simulink model "EHB_MOTOR"  (R2023b)
settings: Solver=FixedStepDiscrete  StartTime=0.0  StopTime=inf  FixedStep=0.0001  RelTol=1e-3  EnableMultiTasking=on
undefined symbols (not defined in the file): CAN_EHB_VCU0x125, CAN_EHB_VCU0x126, CAN_id0x120_Data, Cos_Table, Cos_Table1, EHB_DTC_status, R, Sin_BreakPoint, Sin_BreakPoint1, Sin_Table, Sin_Table1, T
libraries: simulink x30
(part 9 of 9)

== stateflow chart EHB_MOTOR/EHB_MOTOR_PRO/INPUT/DI/Debounce7 ==
  state none
    en:cnt_0=0;
    cnt_1=0;
    none -> (junction 63)
    (junction 63) -> (junction 49) [order 1] : [input>0]
    (junction 63) -> (junction 58) [order 2]
    (junction 49) -> (junction 60)
    (junction 58) -> (junction 62) [order 1] : [cnt_0>=2]
    (junction 60) -> (junction 54) [order 1] : [cnt_1>=2]
    (junction 62) -> (junction 47) : {output=0;
        | cnt_0=0;
        | cnt_1=0;}
    (junction 58) -> (junction 68) [order 2] : {cnt_0=cnt_0+1;}
    (junction 60) -> (junction 66) [order 2] : {cnt_1=cnt_1+1;}
    (junction 54) -> (junction 56) : {output=1;
        | cnt_0=0;
        | cnt_1=0;}
    (junction 47) -> (junction 68)
    (junction 66) -> (junction 68)
    (junction 56) -> (junction 66)
  (default) -> none
  data: cnt_0 local uint8 size=1; output output boolean size=1; input input; cnt_1 local uint8 size=1

== stateflow chart EHB_MOTOR/EHB_MOTOR_PRO/INPUT/DI/Debounce8 ==
  state none
    en:cnt_0=0;
    cnt_1=0;
    none -> (junction 63)
    (junction 63) -> (junction 49) [order 1] : [input>0]
    (junction 63) -> (junction 58) [order 2]
    (junction 49) -> (junction 60)
    (junction 58) -> (junction 62) [order 1] : [cnt_0>=2]
    (junction 60) -> (junction 54) [order 1] : [cnt_1>=2]
    (junction 62) -> (junction 47) : {output=0;
        | cnt_0=0;
        | cnt_1=0;}
    (junction 58) -> (junction 68) [order 2] : {cnt_0=cnt_0+1;}
    (junction 60) -> (junction 66) [order 2] : {cnt_1=cnt_1+1;}
    (junction 54) -> (junction 56) : {output=1;
        | cnt_0=0;
        | cnt_1=0;}
    (junction 47) -> (junction 68)
    (junction 66) -> (junction 68)
    (junction 56) -> (junction 66)
  (default) -> none
  data: cnt_0 local uint8 size=1; output output boolean size=1; input input; cnt_1 local uint8 size=1

== stateflow chart EHB_MOTOR/EHB_MOTOR_PRO/INPUT/DI/Debounce9 ==
  state none
    en:cnt_0=0;
    cnt_1=0;
    none -> (junction 63)
    (junction 63) -> (junction 49) [order 1] : [input>0]
    (junction 63) -> (junction 58) [order 2]
    (junction 49) -> (junction 60)
    (junction 58) -> (junction 62) [order 1] : [cnt_0>=2]
    (junction 60) -> (junction 54) [order 1] : [cnt_1>=2]
    (junction 62) -> (junction 47) : {output=0;
        | cnt_0=0;
        | cnt_1=0;}
    (junction 58) -> (junction 68) [order 2] : {cnt_0=cnt_0+1;}
    (junction 60) -> (junction 66) [order 2] : {cnt_1=cnt_1+1;}
    (junction 54) -> (junction 56) : {output=1;
        | cnt_0=0;
        | cnt_1=0;}
    (junction 47) -> (junction 68)
    (junction 66) -> (junction 68)
    (junction 56) -> (junction 66)
  (default) -> none
  data: cnt_0 local uint8 size=1; output output boolean size=1; input input; cnt_1 local uint8 size=1

== stateflow chart EHB_MOTOR/EHB_MOTOR_PRO/INPUT/AI/EHB_interface/12vADC2VOLT/Filter/Chart ==
  (default) -> (junction 44)
  (junction 44) -> (junction 41) : {i=0;}
  (junction 41) -> (junction 37) [order 1] : [i<Filter_C]
  (junction 36) -> (junction 41) : {i=i+1;}
  (junction 37) -> (junction 36) : {Filter_Input[i]=Filter_Input[i+1];
      | Filter_Input[Filter_C]=input;
      | sum=sum+Filter_Input[i];
      | output=sum/Filter_C;}
  (junction 41) -> (junction 38) [order 2] : {sum=0;}
  data: input input; output output; i local uint8; Filter_C input uint8; sum local double; Filter_Input local double size=20

== stateflow chart EHB_MOTOR/EHB_MOTOR_PRO/INPUT/AI/EHB_interface/12vLogic2VOLT/Filter/Chart ==
  (default) -> (junction 44)
  (junction 44) -> (junction 41) : {i=0;}
  (junction 41) -> (junction 37) [order 1] : [i<Filter_C]
  (junction 36) -> (junction 41) : {i=i+1;}
  (junction 37) -> (junction 36) : {Filter_Input[i]=Filter_Input[i+1];
      | Filter_Input[Filter_C]=input;
      | sum=sum+Filter_Input[i];
      | output=sum/Filter_C;}
  (junction 41) -> (junction 38) [order 2] : {sum=0;}
  data: input input; output output; i local uint8; Filter_C input uint8; sum local double; Filter_Input local double size=20

== stateflow chart EHB_MOTOR/EHB_MOTOR_PRO/INPUT/AI/EHB_interface/5vADC2VOLT/Filter/Chart ==
  (default) -> (junction 44)
  (junction 44) -> (junction 41) : {i=0;}
  (junction 41) -> (junction 37) [order 1] : [i<Filter_C]
  (junction 36) -> (junction 41) : {i=i+1;}
  (junction 37) -> (junction 36) : {Filter_Input[i]=Filter_Input[i+1];
      | Filter_Input[Filter_C]=input;
      | sum=sum+Filter_Input[i];
      | output=sum/Filter_C;}
  (junction 41) -> (junction 38) [order 2] : {sum=0;}
  data: input input; output output; i local uint8; Filter_C input uint8; sum local double; Filter_Input local double size=20

== stateflow chart EHB_MOTOR/EHB_MOTOR_PRO/INPUT/AI/EHB_interface/Reserve/Filter/Chart ==
  (default) -> (junction 44)
  (junction 44) -> (junction 41) : {i=0;}
  (junction 41) -> (junction 37) [order 1] : [i<Filter_C]
  (junction 36) -> (junction 41) : {i=i+1;}
  (junction 37) -> (junction 36) : {Filter_Input[i]=Filter_Input[i+1];
      | Filter_Input[Filter_C]=input;
      | sum=sum+Filter_Input[i];
      | output=sum/Filter_C;}
  (junction 41) -> (junction 38) [order 2] : {sum=0;}
  data: input input; output output; i local uint8; Filter_C input uint8; sum local double; Filter_Input local double size=20

== stateflow chart EHB_MOTOR/EHB_MOTOR_PRO/INPUT/AI/EHB_interface/VpreADC2Pressure/Filter/Chart ==
  (default) -> (junction 44)
  (junction 44) -> (junction 41) : {i=0;}
  (junction 41) -> (junction 37) [order 1] : [i<Filter_C]
  (junction 36) -> (junction 41) : {i=i+1;}
  (junction 37) -> (junction 36) : {Filter_Input[i]=Filter_Input[i+1];
      | Filter_Input[Filter_C]=input;
      | sum=sum+Filter_Input[i];
      | output=sum/Filter_C;}
  (junction 41) -> (junction 38) [order 2] : {sum=0;}
  data: input input; output output; i local uint8; Filter_C input uint8; sum local double; Filter_Input local double size=20

== stateflow chart EHB_MOTOR/EHB_MOTOR_PRO/INPUT/AI/EHB_interface/KL15ADC2VOLT/Filter/Chart ==
  (default) -> (junction 44)
  (junction 44) -> (junction 41) : {i=0;}
  (junction 41) -> (junction 37) [order 1] : [i<Filter_C]
  (junction 36) -> (junction 41) : {i=i+1;}
  (junction 37) -> (junction 36) : {Filter_Input[i]=Filter_Input[i+1];
      | Filter_Input[Filter_C]=input;
      | sum=sum+Filter_Input[i];
      | output=sum/Filter_C;}
  (junction 41) -> (junction 38) [order 2] : {sum=0;}
  data: input input; output output; i local uint8; Filter_C input uint8; sum local double; Filter_Input local double size=20

== stateflow chart EHB_MOTOR/EHB_MOTOR_PRO/INPUT/AI/EHB_interface/UADC2Cur/Filter/Chart ==
  (default) -> (junction 44)
  (junction 44) -> (junction 41) : {i=0;}
  (junction 41) -> (junction 37) [order 1] : [i<Filter_C]
  (junction 36) -> (junction 41) : {i=i+1;}
  (junction 37) -> (junction 36) : {Filter_Input[i]=Filter_Input[i+1];
      | Filter_Input[Filter_C]=input;
      | sum=sum+Filter_Input[i];
      | output=sum/Filter_C;}
  (junction 41) -> (junction 38) [order 2] : {sum=0;}
  data: input input; output output; i local uint8; Filter_C input uint8; sum local double; Filter_Input local double size=20
